simulink model "H634"  (Simulink 7.3)
settings: Solver=ode45  StartTime=0.001  StopTime=6  RelTol=1e-5
libraries: simulink x6
settings Model: Creator=AlexHomeLab  LastModifiedBy=Sainquake Notebook

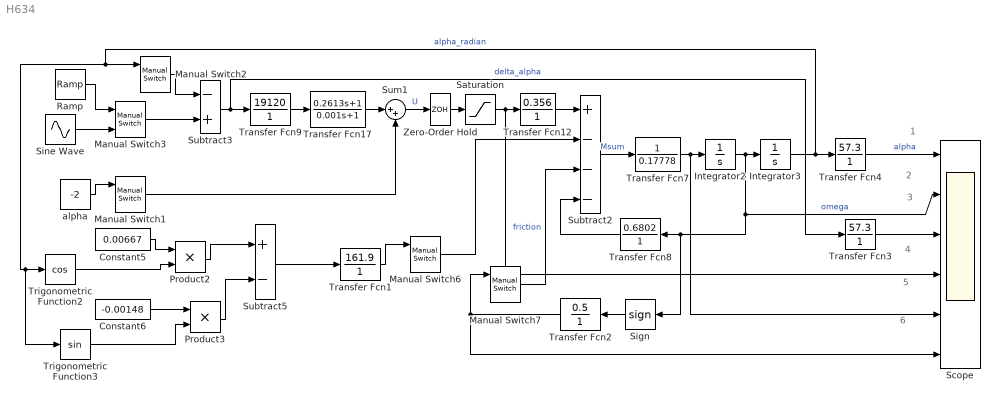
== system H634 ==
  note: 1
  note: 2
  note: 3
  note: 4
  note: 5
  note: 6
  Constant5 : Constant  Value=0.00667
  Constant6 : Constant  Value=-0.00148
  Integrator2 : Integrator
  Integrator3 : Integrator
  Manual Switch1 : simulink/Signal Routing/Manual Switch  SystemSampleTime=-1  sw=1  action=0  varsize=off
  Manual Switch2 : simulink/Signal Routing/Manual Switch  SystemSampleTime=-1  sw=1  action=0  varsize=off
  Manual Switch3 : simulink/Signal Routing/Manual Switch  SystemSampleTime=-1  sw=0  action=0  varsize=off
  Manual Switch6 : simulink/Signal Routing/Manual Switch  SystemSampleTime=-1  sw=1  action=0  varsize=off
  Manual Switch7 : simulink/Signal Routing/Manual Switch  SystemSampleTime=-1  sw=0  action=0  varsize=off
  Product2 : Product  RndMeth=Zero
  Product3 : Product  RndMeth=Zero
  Ramp : simulink/Sources/Ramp  SystemSampleTime=-1  slope=0.5  start=0  X0=0
  Saturation : Saturate  UpperLimit=27  LowerLimit=-27
  Scope : Scope  NumInputPorts=6
      settings: YMin=-30~-1.5~-0.1~-30~-75~-0.2  YMax=30~1.5~0.6~30~75~0.2  MaxDataPoints=5000000
  Sign : Signum
  Sine Wave : Sin  Amplitude=0.5  Bias=0  Frequency=2  Phase=0  Samples=10  SampleTime=0  Offset=0
  Subtract2 : Sum  Inputs=+---
  Subtract3 : Sum  Inputs=-+
  Subtract5 : Sum  Inputs=+-
  Sum1 : Sum  Inputs=|++
  Transfer Fcn1 : TransferFcn  Numerator=[161.9]  Denominator=[ 1 ]
  Transfer Fcn12 : TransferFcn  Numerator=[0.356]  Denominator=[ 1 ]
  Transfer Fcn17 : TransferFcn  Numerator=[0.2613 1]  Denominator=[0.001 1]
  Transfer Fcn2 : TransferFcn  Numerator=[0.5]  Denominator=[ 1 ]
  Transfer Fcn3 : TransferFcn  Numerator=[57.3]  Denominator=[ 1 ]
  Transfer Fcn4 : TransferFcn  Numerator=[57.3]  Denominator=[ 1 ]
  Transfer Fcn7 : TransferFcn  Denominator=0.17778
  Transfer Fcn8 : TransferFcn  Numerator=[0.6802]  Denominator=[ 1]
  Transfer Fcn9 : TransferFcn  Numerator=[19120]  Denominator=[ 1 ]
  Trigonometric Function2 : Trigonometry  Operator=cos
  Trigonometric Function3 : Trigonometry
  Zero-Order Hold : ZeroOrderHold  SampleTime=1/19531
  alpha : Constant  Value=-2
  wires:
  Subtract2/1 -> Transfer Fcn7/1  "Msum"
  Integrator2/1 -> Integrator3/1, Transfer Fcn8/1, Sign/1, Scope/2  "omega"
  Transfer Fcn7/1 -> Integrator2/1, Scope/5
  Integrator3/1 -> Transfer Fcn4/1, Trigonometric Function2/1, Trigonometric Function3/1, Manual Switch2/1  "alpha_radian"
  Subtract3/1 -> Transfer Fcn3/1, Transfer Fcn9/1  "delta_alpha"
  Transfer Fcn8/1 -> Subtract2/4
  Transfer Fcn12/1 -> Subtract2/1
  Transfer Fcn9/1 -> Transfer Fcn17/1
  Constant5/1 -> Product2/1
  Trigonometric Function2/1 -> Product2/2
  Constant6/1 -> Product3/1
  Trigonometric Function3/1 -> Product3/2
  Product3/1 -> Subtract5/2
  Product2/1 -> Subtract5/1
  Subtract5/1 -> Transfer Fcn1/1
  Manual Switch6/1 -> Subtract2/2
  Transfer Fcn17/1 -> Sum1/1
  Transfer Fcn1/1 -> Manual Switch6/1
  Manual Switch7/1 -> Subtract2/3  "friction"
  alpha/1 -> Manual Switch1/1
  Transfer Fcn4/1 -> Scope/1  "alpha"
  Manual Switch2/1 -> Subtract3/1
  Transfer Fcn3/1 -> Scope/3
  Saturation/1 -> Transfer Fcn12/1, Scope/4
  Manual Switch1/1 -> Sum1/2
  Sign/1 -> Transfer Fcn2/1
  Transfer Fcn2/1 -> Manual Switch7/1, Scope/6
  Zero-Order Hold/1 -> Saturation/1
  Sum1/1 -> Zero-Order Hold/1  "U"
  Ramp/1 -> Manual Switch3/1
  Sine Wave/1 -> Manual Switch3/2
  Manual Switch3/1 -> Subtract3/2
